simulink model "differential_drive"  (R2018a)
settings: Solver=VariableStepAuto  StartTime=0.0  StopTime=inf  FixedStep=0.7  MaxStep=0.1  RelTol=1e-3
libraries: simulink x3
settings Model: EnablePacing=on  Creator=U500304  LastModifiedBy=U500304

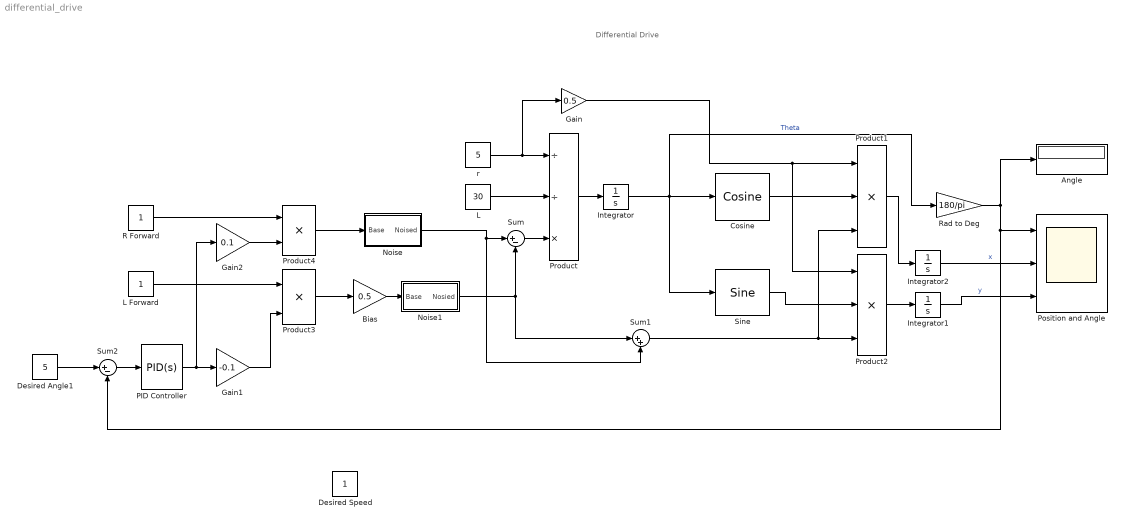
== system differential_drive ==
  note: Differential Drive
  Angle : Display
      settings: AttributesFormatString=Degrees
  Bias : Gain  Gain=0.5
  Cosine : simulink/Lookup Tables/Cosine  Formula=cos(2*pi*u)  NumDataPoints=(2^5)+1  OutputWordLength=16  InternalRulePriority=Speed
      settings: SourceProductName=Simulink  SourceProductBaseCode=SL
  Desired Angle1 : Constant  Value=5
  Desired Speed : Constant
  Gain : Gain  Gain=0.5
  Gain1 : Gain  Gain=-0.1
  Gain2 : Gain  Gain=0.1
  Integrator : Integrator
  Integrator1 : Integrator
  Integrator2 : Integrator
  L : Constant  Value=30
  L Forward : Constant
  Noise : Subsystem
  Noise1 : Subsystem
  PID Controller : simulink/Continuous/PID Controller  Controller=PID  TimeDomain=Continuous-time  SampleTime=-1  IntegratorMethod=Forward Euler  FilterMethod=Forward Euler  Form=Parallel  UseFilter=on  ControllerParametersSource=internal  P=200  I=100  D=1  N=1  InitialConditionSource=internal  InitialConditionForIntegrator=0  InitialConditionForFilter=0  ExternalReset=none  LimitOutput=off  UpperSaturationLimit=inf  LowerSaturationLimit=-inf  LinearizeAsGain=on  AntiWindupMode=none  Kb=1  TrackingMode=off  Kt=1  PParamMin=[]  PParamMax=[]  IParamMin=[]  IParamMax=[]  DParamMin=[]  DParamMax=[]  NParamMin=[]  NParamMax=[]  KbParamMin=[]  KbParamMax=[]  KtParamMin=[]  KtParamMax=[]  POutMin=[]  POutMax=[]  IOutMin=[]  IOutMax=[]  DOutMin=[]  DOutMax=[]  NOutMin=[]  NOutMax=[]  KbOutMin=[]  KbOutMax=[]  KtOutMin=[]  KtOutMax=[]  IntegratorOutMin=[]  IntegratorOutMax=[]  FilterOutMin=[]  FilterOutMax=[]  SumOutMin=[]  SumOutMax=[]  SumI1OutMin=[]  SumI1OutMax=[]  SumI2OutMin=[]  SumI2OutMax=[]  SumI3OutMin=[]  SumI3OutMax=[]  SumDOutMin=[]  SumDOutMax=[]  SaturationOutMin=[]  SaturationOutMax=[]  IntegratorContinuousStateAttributes=''  IntegratorStateMustResolveToSignalObject=off  IntegratorRTWStateStorageClass=Auto  FilterContinuousStateAttributes=''  FilterStateMustResolveToSignalObject=off  FilterRTWStateStorageClass=Auto  DifferentiatorICPrevScaledInput=0  DifferentiatorOutMin=[]  DifferentiatorOutMax=[]  FilterDiffOutCoefMin=[]  FilterDiffOutCoefMax=[]  SumDenOutMin=[]  SumDenOutMax=[]  SumNumOutMin=[]  SumNumOutMax=[]  ReciprocalOutMin=[]  ReciprocalOutMax=[]  DivideOutMin=[]  DivideOutMax=[]  TunerSelectOption=Transfer Function Based (PID Tuner App)
  Position and Angle : Scope  NumInputPorts=3
  Product : Product  Inputs=//*
  Product1 : Product  Inputs=3
  Product2 : Product  Inputs=3
  Product3 : Product
  Product4 : Product
  R Forward : Constant
  Rad to Deg : Gain  Gain=180/pi
  Sine : simulink/Lookup Tables/Sine  Formula=sin(2*pi*u)  NumDataPoints=(2^5)+1  OutputWordLength=16  InternalRulePriority=Speed
      settings: SourceProductName=Simulink
  Sum : Sum  Inputs=|+-
  Sum1 : Sum  Inputs=|++
  Sum2 : Sum  Inputs=|+-
  r : Constant  Value=5
  wires:
  Product1/1 -> Integrator2/1
  Product2/1 -> Integrator1/1
  Rad to Deg/1 -> Sum2/2, Position and Angle/1, Angle/1
  Noise1/1(Nosied) -> Sum1/1, Sum/2
  Sum/1 -> Product/3
  r/1 -> Gain/1, Product/1
  L/1 -> Product/2
  Product/1 -> Integrator/1
  Integrator/1 -> Cosine/1, Rad to Deg/1, Sine/1  "Theta"
  Sum1/1 -> Product1/3, Product2/3
  Gain/1 -> Product1/1, Product2/1
  Cosine/1 -> Product1/2
  Sine/1 -> Product2/2
  Integrator1/1 -> Position and Angle/3  "y"
  Integrator2/1 -> Position and Angle/2  "x"
  Sum2/1 -> PID Controller/1
  L Forward/1 -> Product3/1
  Desired Angle1/1 -> Sum2/1
  Product3/1 -> Bias/1
  PID Controller/1 -> Gain2/1, Gain1/1
  Gain1/1 -> Product3/2
  Noise/1(Noised) -> Sum1/2, Sum/1
  R Forward/1 -> Product4/1
  Gain2/1 -> Product4/2
  Product4/1 -> Noise/1(Base)
  Bias/1 -> Noise1/1(Base)

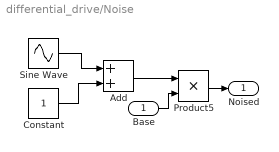
== system differential_drive/Noise ==
  Base : Inport
  Add : Sum
  Constant : Constant
  Product5 : Product
  Sine Wave : Sin  Amplitude=0.07  SampleTime=0
  Noised : Outport
  wires:
  Add/1 -> Product5/1
  Sine Wave/1 -> Add/1
  Base/1 -> Product5/2
  Constant/1 -> Add/2
  Product5/1 -> Noised/1

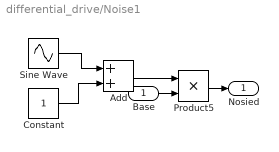
== system differential_drive/Noise1 ==
  Base : Inport
  Add : Sum
  Constant : Constant
  Product5 : Product
  Sine Wave : Sin  Amplitude=0.07  SampleTime=0
  Nosied : Outport
  wires:
  Product5/1 -> Nosied/1
  Constant/1 -> Add/2
  Base/1 -> Product5/2
  Sine Wave/1 -> Add/1
  Add/1 -> Product5/1
